simulink model "task1_nonlin_model_simu"  (R2017b)
settings: Solver=VariableStepAuto  StartTime=0.0  StopTime=10.0  RelTol=1e-3
values from neighbouring files (symbols this model uses):
  alpha = [alpha1; alpha2]    [OAC_LA_Ass2.m]    (also in testfile.m)
  beta = [beta1; beta2]    [OAC_LA_Ass2.m]    (also in testfile.m)
  gamma = [gamma1; gamma2]    [OAC_LA_Ass2.m]    (also in testfile.m)
  k = [k1; k2]    [OAC_LA_Ass2.m]    (also in testfile.m)
  x0 = x_eq    [OAC_LA_Ass2.m]    (also in testfile.m = [xe(1); xe(2)])
settings Model: Creator=miko2  LastModifiedBy=lukastotschnig

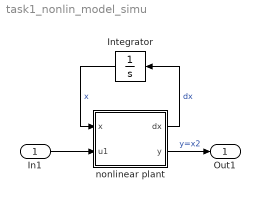
== system task1_nonlin_model_simu ==
  In1 : Inport
  Integrator : Integrator  InitialCondition=x0
  nonlinear plant : MATLAB Function  TreatAsAtomicUnit=on
  Out1 : Outport
  wires:
  nonlinear plant/1(dx) -> Integrator/1  "dx"
  Integrator/1 -> nonlinear plant/1(x)  "x"
  nonlinear plant/2(y) -> Out1/1  "y=x2"
  In1/1 -> nonlinear plant/2(u1)

== matlab function task1_nonlin_model_simu/nonlinear plant ==
  data: dx output; x input; y output; u1 input; k parameter; alpha parameter; beta parameter; gamma parameter
function [dx,y] = fcn(x,u1,k,alpha, beta, gamma)
    
    % calculate input quantity
    if (beta(1)+gamma(1)*u1) <= 0
        zp1 = 0;
    else
        zp1 = alpha(1) + sqrt( beta(1)+gamma(1)*u1 );
    end
    
    % nonlinear plant description
   dx1 = -k(1)*sqrt(x(1)) + zp1;
   dx2 = -k(2)*sqrt(x(2)) + k(1)*sqrt(x(1));
   
   dx = [dx1; dx2];
   y = x(2);

end
